simulink model "Assignment1"  (R2021a)
settings: Solver=FixedStepAuto  StartTime=0.0  StopTime=10.0  FixedStep=1e-4  RelTol=1e-3  EnableMultiTasking=on
undefined symbols (not defined in the file): D0, D1, PTC16, PTC17
libraries: frdmk64flib x4
settings Model: EnablePacing=on  PacingRate=0.250000  ExtModeTrigDuration=5  Creator=Arun Mistry  LastModifiedBy=Arun Mistry
settings OptimizationCC: EnhancedBackFolding=on  PassReuseOutputArgsAs=Individual arguments  ZeroExternalMemoryAtStartup=off  ZeroInternalMemoryAtStartup=off  MaxStackSize=64  OptimizeBlockOrder=speed  DifferentSizesBufferReuse=on  OptimizationCustomize=off  EfficientTunableParamExpr=on
settings DebuggingCC: ParameterTunabilityLossMsg=error
settings HardwareCC: ProdBitPerPointer=32  ProdBitPerSizeT=32  ProdBitPerPtrDiffT=32  ProdLargestAtomicInteger=Long  ProdLargestAtomicFloat=Double  ProdWordSize=32  ProdHWDeviceType=ARM Compatible->ARM Cortex
settings SFSimCC: MATLABDynamicMemAlloc=off
settings RTWCC: SystemTargetFile=ert.tlc  HardwareBoard=NXP FRDM-K64F  TLCOptions="-aInlineSetEventsForThisBaseRateFcn=TLC_FALSE -aSuppressMultiTaskScheduler=TLC_FALSE  -aRateBasedStepFcn=0"  TemplateMakefile=ert_default_tmf  Toolchain=GNU Tools for ARM Embedded Processors
settings CodeAppCC: ForceParamTrailComments=on  IgnoreCustomStorageClasses=off  OperatorAnnotations=on  SimulinkDataObjDesc=on  SFDataObjDesc=on  InsertBlockDesc=on
settings ERTTargetCC: ExtModeTransport=4  ExtModeMexFile=sendToCommService

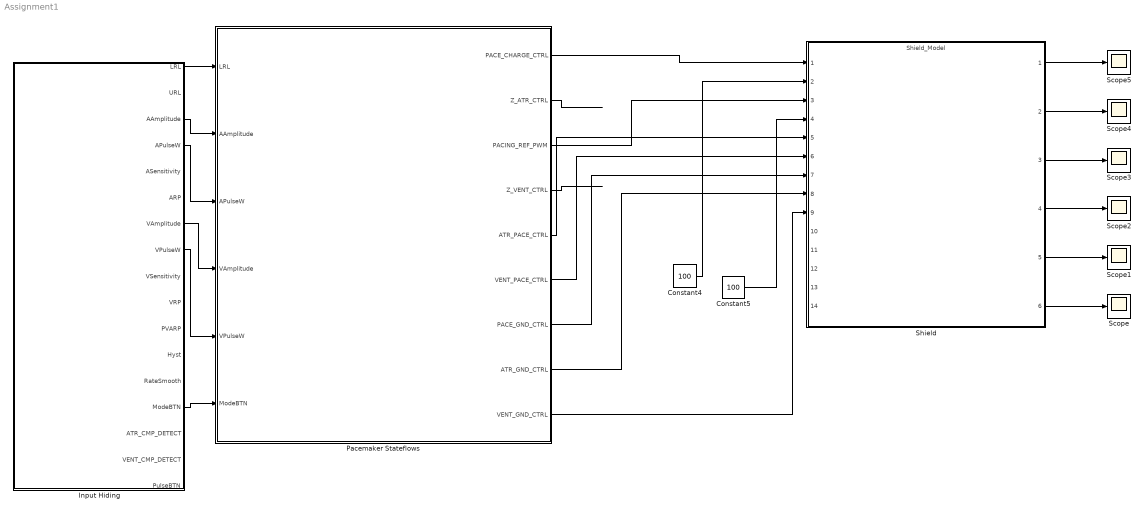
== system Assignment1 ==
  Constant4 : Constant  Value=100
  Constant5 : Constant  Value=100
  Input Hiding : Subsystem
  Pacemaker Stateflows : Stateflow chart  TreatAsAtomicUnit=on
  Scope{,1..5} (6 alike) : Scope
  Shield : ModelReference  ModelNameDialog=Shield_Model.slxp  ModelReferenceVersion=1.25  CopyOfModelProtected=on
  wires:
  Input Hiding/1(LRL) -> Pacemaker Stateflows/1(LRL)
  Input Hiding/8(VPulseW) -> Pacemaker Stateflows/5(VPulseW)
  Input Hiding/4(APulseW) -> Pacemaker Stateflows/3(APulseW)
  Pacemaker Stateflows/4(Z_VENT_CTRL) -> ?
  Input Hiding/3(AAmplitude) -> Pacemaker Stateflows/2(AAmplitude)
  Input Hiding/7(VAmplitude) -> Pacemaker Stateflows/4(VAmplitude)
  Pacemaker Stateflows/2(Z_ATR_CTRL) -> ?
  Input Hiding/14(ModeBTN) -> Pacemaker Stateflows/6(ModeBTN)
  Shield/2 -> Scope4/1
  Constant5/1 -> Shield/4
  Constant4/1 -> Shield/2
  Shield/6 -> Scope/1
  Shield/1 -> Scope5/1
  Pacemaker Stateflows/6(VENT_PACE_CTRL) -> Shield/6
  Pacemaker Stateflows/5(ATR_PACE_CTRL) -> Shield/5
  Pacemaker Stateflows/1(PACE_CHARGE_CTRL) -> Shield/1
  Shield/3 -> Scope3/1
  Shield/4 -> Scope2/1
  Shield/5 -> Scope1/1
  Pacemaker Stateflows/3(PACING_REF_PWM) -> Shield/3
  Pacemaker Stateflows/8(ATR_GND_CTRL) -> Shield/8
  Pacemaker Stateflows/7(PACE_GND_CTRL) -> Shield/7
  Pacemaker Stateflows/9(VENT_GND_CTRL) -> Shield/9

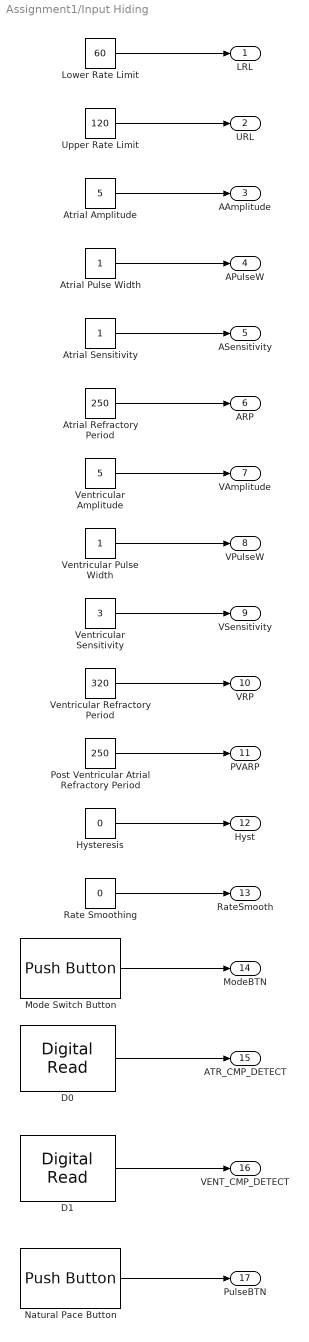
== system Assignment1/Input Hiding ==
  Atrial Amplitude : Constant  Value=5
  Atrial Pulse Width : Constant
  Atrial Refractory Period : Constant  Value=250
  Atrial Sensitivity : Constant
  D0 : frdmk64flib/Digital Read  Whichpin=PTC16 (D0)  SampleTime=-1
  D1 : frdmk64flib/Digital Read  Whichpin=PTC17 (D1)  SampleTime=-1
  Hysteresis : Constant  Value=0
  Lower Rate Limit : Constant  Value=60
  Mode Switch Button : frdmk64flib/Push Button  Whichswitch=SW2  SampleTime1=-1
  Natural Pace Button : frdmk64flib/Push Button  Whichswitch=SW3  SampleTime1=-1
  Post Ventricular Atrial Refractory Period : Constant  Value=250
  Rate Smoothing : Constant  Value=0
  Upper Rate Limit : Constant  Value=120
  Ventricular Amplitude : Constant  Value=5
  Ventricular Pulse Width : Constant
  Ventricular Refractory Period : Constant  Value=320
  Ventricular Sensitivity : Constant  Value=3
  LRL : Outport
  URL : Outport  Port=2
  AAmplitude : Outport  Port=3
  APulseW : Outport  Port=4
  ASensitivity : Outport  Port=5
  ARP : Outport  Port=6
  VAmplitude : Outport  Port=7
  VPulseW : Outport  Port=8
  VSensitivity : Outport  Port=9
  VRP : Outport  Port=10
  PVARP : Outport  Port=11
  Hyst : Outport  Port=12
  RateSmooth : Outport  Port=13
  ModeBTN : Outport  Port=14
  ATR_CMP_DETECT : Outport  Port=15
  VENT_CMP_DETECT : Outport  Port=16
  PulseBTN : Outport  Port=17
  wires:
  Lower Rate Limit/1 -> LRL/1
  Upper Rate Limit/1 -> URL/1
  Atrial Amplitude/1 -> AAmplitude/1
  Ventricular Amplitude/1 -> VAmplitude/1
  Atrial Pulse Width/1 -> APulseW/1
  Ventricular Pulse Width/1 -> VPulseW/1
  Atrial Sensitivity/1 -> ASensitivity/1
  Ventricular Sensitivity/1 -> VSensitivity/1
  Ventricular Refractory Period/1 -> VRP/1
  Atrial Refractory Period/1 -> ARP/1
  D1/1 -> VENT_CMP_DETECT/1
  D0/1 -> ATR_CMP_DETECT/1
  Post Ventricular Atrial Refractory Period/1 -> PVARP/1
  Hysteresis/1 -> Hyst/1
  Rate Smoothing/1 -> RateSmooth/1
  Mode Switch Button/1 -> ModeBTN/1
  Natural Pace Button/1 -> PulseBTN/1

== stateflow chart Assignment1/Pacemaker Stateflows ==
  state AOO
    state ENTRY
      entry:
      VENT_PACE_CTRL = 0; VENT_GND_CTRL = 0; PACE_GND_CTRL = 1;
      Z_VENT_CTRL = false; Z_ATR_CTRL = false; PACING_REF_PWM = AAmplitude*20;
    state PACE_ATR
      entry:
      PACE_CHARGE_CTRL = 0;
      ATR_GND_CTRL = 0;
      ATR_PACE_CTRL = 1;
    state C22_CHARGE
      entry:
      ATR_PACE_CTRL = 0;
      ATR_GND_CTRL = 1;
      PACE_CHARGE_CTRL = 1;
    (default) -> AOO.ENTRY
    AOO.ENTRY -> AOO.C22_CHARGE
    PACE_ATR -> AOO.C22_CHARGE : after(APulseW,msec)
    AOO.C22_CHARGE -> PACE_ATR : after((60000/LRL)-APulseW,msec)
  state VOO
    state ENTRY
      entry:
      ATR_PACE_CTRL = 0; ATR_GND_CTRL = 0; PACE_GND_CTRL = 1;
      Z_ATR_CTRL = false; Z_VENT_CTRL = false; PACING_REF_PWM = VAmplitude*20;
    state PACE_VENT
      entry:
      PACE_CHARGE_CTRL = 0;
      VENT_GND_CTRL = 0;
      VENT_PACE_CTRL = 1;
    state C22_CHARGE
      entry:
      VENT_PACE_CTRL = 0;
      VENT_GND_CTRL = 1;
      PACE_CHARGE_CTRL = 1;
    (default) -> VOO.ENTRY
    VOO.ENTRY -> VOO.C22_CHARGE
    PACE_VENT -> VOO.C22_CHARGE : after(VPulseW,msec)
    VOO.C22_CHARGE -> PACE_VENT : after((60000/LRL)-VPulseW,msec)
  state MODE
    entry:
    Mode = Mode + 1;
    Mode = rem(Mode ,4);
  state AAI
  state VVI
  (default) -> MODE
  MODE -> VOO [order 2] : [Mode==1&&ModeBTN==false]
  MODE -> AOO [order 1] : [Mode==0&&ModeBTN==false]
  VOO -> MODE : [ModeBTN==true]
  AOO -> MODE : [ModeBTN==true]
  AAI -> MODE : [ModeBTN==true]
  MODE -> AAI [order 3] : [Mode==2&&ModeBTN==false]
  VVI -> MODE : [ModeBTN==true]
  MODE -> VVI [order 4] : [Mode==3&&ModeBTN==false]
  data: LRL input; AAmplitude input; APulseW input; VAmplitude input; VPulseW input; PACE_CHARGE_CTRL output; Z_ATR_CTRL output; PACING_REF_PWM output; Z_VENT_CTRL output; ATR_PACE_CTRL output; VENT_PACE_CTRL output; PACE_GND_CTRL output; ATR_GND_CTRL output; VENT_GND_CTRL output; ModeBTN input; Mode local =3
